simulink model "VehicleDynamicsModel"  (R2018a)
settings: Solver=ode15s  StartTime=0.0  StopTime=12  FixedStep=0.01  RelTol=1e-2  EnableMultiTasking=on
PreLoadFcn:
  | PowerTrain_14DOF_ini
StopFcn:
  | AfterSim
undefined symbols (not defined in the file): AccelCmd2TrqCmd, Chasis, GearRatio, Motor, Motor_J, Motor_RotorDamping, VEH, X, Y, Z
libraries: sm_lib x186, autolibutils x40, nesl_utility x23, vehdynlibtire x4, fuzblock x3, sharedtransform x2, autolibmappedmotorcommon x2, vehdynlibeom x1, vehdynlibsuspension x1, simulink x1, vehdynlibsteering x1
(part 5 of 11)

== system VehicleDynamicsModel/E23/PowerTrain/PowerTrain/MotorRL/Motor/Motor ==
  TrqCmd : Inport
  BattVolt : Inport  Port=2
  MtrSpd : Inport  Port=3
  Bus Creator : BusCreator  Inputs=3
  Bus Selector : BusSelector  OutputSignals=signal1.MechPwr,BattCur,MtrTrq
  Divide : Product  Inputs=**
  Mapped Motor : Subsystem  AncestorBlock=autolibmappedmotor/Mapped Motor  mask(MappedMotor){port_config=Speed, param_by=Tabulated torque-speed envelope, w_t=Motor.Motor_n, T_t=Motor.Motor_Tq, torque_max=123, power_max=50, Tc=Motor.Motor_Tc, param_loss=Tabulated efficiency data, eff=96, w_eff=1000, T_eff=120, Piron=0, Pbase=5, w_eff_bp=Motor.Motor_n_e, T_eff_bp=Motor.Motor_Tq_e, losses_table=[1.49 1.67 2.21 3.10; 0.42 0.69 1.14 2.03; 0.06 0.24 0.78 1.68; 0.42 0.69 1.14 2.03; 1.49 1.67 2.21 3.10], efficiency_table=Motor.Motor_efficiency, J=Motor_J, b=Motor_RotorDamping, omega_o=0, T_t_extended=[0 48.13 49.32 50.18 50.79 51.89 53.34 54.25 55.67 57.12 58.37 60.15 61.25 63.29 65.1 66.47 68.15 70.26 72.09 75.05 77 80.33 82 85.17 88.15 92.06 96.45 99.14 104.15 109.88 114.54 119.13 120.12 120.08 120.05 120 120.16 120.38 120.32 120.12 120.03 120.29 120.06 120.09 120.09 120 120.12 120.08 120.17 120.13 120.02 120.13 120.17 120.08 120.12 120 120.09 120.09 120.06 120.29 120.03 120.12 120.32 120.38 120.16 120 120.05 120.08 120.12 119.13 114.54 109.88 104.15 99.14 96.45 92.06 88.15 85.17 82 80.33 77 75.05 72.09 70.26 68.15 66.47 65.1 63.29 61.25 60.15 58.37 57.12 55.67 54.25 53.34 51.89 50.79 50.18 49.32 48.13 0], w_t_extended=[-1047.1975511966 -1026.14888041755 -1005.30964914873 -984.365698124802 -963.42174710087 -942.373076321818 -921.533845053006 -900.485174273954 -879.645943005142 -858.70199198121 -837.758040957278 -816.918809688466 -795.870138909414 -774.821468130363 -753.877517106431 -733.038285837618 -712.094334813686 -691.150383789755 -670.206432765823 -649.26248174189 -628.318530717959 -607.374579694027 -586.325908914975 -565.486677646163 -544.542726622231 -523.598775598299 -502.550104819247 -481.710873550435 -460.766922526503 -439.718251747451 -418.879020478639 -416.784625376246 -397.935069454707 -376.886398675656 -356.151887161963 -335.103216382911 -314.159265358979 -293.215314335047 -251.327412287183 -230.383461263251 -209.43951023932 -188.495559215388 -167.551608191456 -146.607657167524 -125.663706143592 -104.71975511966 -83.7758040957278 -62.8318530717959 -41.8879020478639 -20.943951023932 0 20.943951023932 41.8879020478639 62.8318530717959 83.7758040957278 104.71975511966 125.663706143592 146.607657167524 167.551608191456 188.495559215388 209.43951023932 230.383461263251 251.327412287183 293.215314335047 314.159265358979 335.103216382911 356.151887161963 376.886398675656 397.935069454707 416.784625376246 418.879020478639 439.718251747451 460.766922526503 481.710873550435 502.550104819247 523.598775598299 544.542726622231 565.486677646163 586.325908914975 607.374579694027 628.318530717959 649.26248174189 670.206432765823 691.150383789755 712.094334813686 733.038285837618 753.877517106431 774.821468130363 795.870138909414 816.918809688466 837.758040957278 858.70199198121 879.645943005142 900.485174273954 921.533845053006 942.373076321818 963.42174710087 984.365698124802 1005.30964914873 1026.14888041755 1047.1975511966], KLossIron=0, KLossCopper=0.34687, x_w_eff_vec=[-1047.1975511966 -1026.25360017267 -1005.30964914873 -984.365698124802 -963.42174710087 -942.477796076938 -921.533845053006 -900.589894029074 -879.645943005142 -858.70199198121 -837.758040957278 -816.814089933346 -795.870138909414 -774.926187885482 -753.98223686155 -733.038285837618 -712.094334813686 -691.150383789755 -670.206432765823 -649.262481741891 -628.318530717959 -607.374579694027 -586.430628670095 -565.486677646163 -544.542726622231 -523.598775598299 -502.654824574367 -481.710873550435 -460.766922526503 -439.822971502571 -418.879020478639 -397.935069454707 -376.991118430775 -356.047167406843 -335.103216382911 -314.159265358979 -293.215314335047 -272.271363311115 -251.327412287183 -230.383461263251 -209.43951023932 -188.495559215388 -167.551608191456 -146.607657167524 -125.663706143592 -104.71975511966 -83.7758040957278 -62.8318530717959 -41.8879020478639 -20.943951023932 0 20.943951023932 41.8879020478639 62.8318530717959 83.7758040957278 104.71975511966 125.663706143592 146.607657167524 167.551608191456 188.495559215388 209.43951023932 230.383461263251 251.327412287183 272.271363311115 293.215314335047 314.159265358979 335.103216382911 356.047167406843 376.991118430775 397.935069454707 418.879020478639 439.822971502571 460.766922526503 481.710873550435 502.654824574367 523.598775598299 544.542726622231 565.486677646163 586.430628670095 607.374579694027 628.318530717959 649.262481741891 670.206432765823 691.150383789755 712.094334813686 733.038285837618 753.98223686155 774.926187885482 795.870138909414 816.814089933346 837.758040957278 858.70199198121 879.645943005142 900.589894029074 921.533845053006 942.477796076938 963.42174710087 984.365698124802 1005.30964914873 1026.25360017267 1047.1975511966], x_T_eff_vec=[-120 -115 -110 -105 -100 -95 -90 -85 -80 -75 -70 -65 -60 -55 -50 -45 -40 -35 -30 -25 -20 -15 -10 -5 0 5 10 15 20 25 30 35 40 45 50 55 60 65 70 75 80 85 90 95 100 105 110 115 120], x_losses_mat=[125538042.437448 120307290.669221 115076538.900994 109845787.132767 104615035.36454 99384283.5963131 94153531.8280861 88922780.0598591 83692028.2916321 78461276.5234051 73230524.7551781 67999772.9869511 62769021.2187241 8077.86936584377 6537.62250747031 5294.23011144442 3494.44036585647 3669.22354297158 2256.0204479155 2432.01617081177 2071.37977159766 1610.62908921637 1294.28910822051 2661.42967385561 0 1764.52787376627 1151.91730631626 1460.84058391925 1884.95559215388 2225.29479629277 2104.86707790516 3335.32420056116 3225.36845768552 4759.51287018854 5811.94640914111 7084.29143384498 62769.0212187241 67999.7729869511 73230.5247551781 78461.2765234051 83692.0282916321 88922.7800598591 94153.5318280861 99384.2835963131 104615.03536454 109845.787132767 115076.538900994 120307.290669221 125538.042437448;123027281.588699 117901144.855837 112775008.122974 107648871.390112 102522734.657249 97396597.9243868 92270461.1915244 87144324.4586619 82018187.7257994 76892050.992937 71765914.2600745 66639777.5272121 61513640.7943496 7478.98291858562 6148.32783978025 4960.79398090109 3813.40135583285 3038.69016103186 2786.66462860407 2322.22052383673 1712.27577926967 1559.72463462365 1426.00158566133 1227.18057517549 0 990.334724166622 1252.02939221065 1416.22996823828 1580.4305442659 2129.47622035828 2555.37146442994 2801.67232847138 3489.26224058706 4479.59696475368 5490.45676092376 6603.9419171111 61513.6407943496 66639.777527212 71765.9142600745 76892.050992937 82018.1877257994 87144.3244586619 92270.4611915244 97396.5979243868 102522.734657249 107648.871390112 112775.008122974 117901.144855837 123027.281588699;120516520.73995 115494999.042452 110473477.344954 105451955.647456 100430433.949959 95408912.2524606 90387390.5549626 85365868.8574647 80344347.1599668 75322825.4624689 70301303.7649709 65279782.067473 60258260.3699751 55236738.6724772 6085.95527511565 4419.61047732237 3213.51680505427 2811.82720442249 2586.95316881922 1949.95406084884 1819.86261459858 1582.94613263751 1255.2235214343 1073.63166413942 0 884.672491250885 1115.89371055509 1432.56625003695 1668.8140175869 1809.55736846772 2382.5838684825 2603.75199129522 2975.71656148025 4026.26514484068 5428.67210540316 55236.7386724772 60258.2603699751 65279.782067473 70301.3037649709 75322.8254624689 80344.3471599668 85365.8688574647 90387.3905549627 95408.9122524606 100430.433949959 105451.955647456 110473.477344954 115494.999042452 120516.52073995;118005759.891201 113088853.229068 108171946.566934 103255039.904801 98338133.2426677 93421226.5805343 88504319.9184009 83587413.2562675 78670506.5941342 73753599.9320008 68836693.2698674 63919786.607734 59002879.9456006 6555.08099423915 5226.72052101664 4009.3848227875 2647.3869362588 2673.06202508028 2394.40304949276 2110.88192594624 1596.26869966184 1424.73982623326 1266.56534521701 958.492286704556 0 802.258043971713 1122.17689586227 1299.36272152474 1476.5485471872 1944.12225379649 2214.8228207808 2480.6015592745 2480.6015592745 3676.60588249613 4724.95535099905 5847.13224686132 59002.8799456006 63919.786607734 68836.6932698674 73753.5999320008 78670.5065941342 83587.4132562676 88504.3199184009 93421.2265805343 98338.1332426677 103255.039904801 108171.946566934 113088.853229068 118005.759891201;115494999.042452 110682707.415683 105870415.788915 101058124.162146 96245832.5353769 91433540.9086081 86621249.2818392 81808957.6550704 76996666.0283015 72184374.4015327 67372082.7747638 62559791.147995 6494.25560337182 6018.70378756779 4590.23504916625 3616.74577866145 2723.1621117198 2694.66773757155 2276.04490415416 1840.76813897098 1517.36326943611 1308.02625424273 1178.59675010095 1036.00029913034 0 852.62824618427 1050.12970433995 1199.46007514058 1406.59575076727 1710.07360110404 2109.8936261509 2495.26232499125 2543.43341234629 3338.25635370451 4190.88459988878 5404.79600123588 5838.33578743127 62559.791147995 67372.0827747638 72184.3744015327 76996.6660283015 81808.9576550704 86621.2492818392 91433.5409086081 96245.8325353769 ...(+77378 chars)], aMode=1}
      mask prompts: port_config "autoblks_shared:autoblkpbgenericelectricmachine:blkPrm_port_config"; param_by "autoblks_shared:autoblkpbgenericelectricmachine:blkPrm_param_by"; w_t "autoblks_shared:autoblkpbgenericelectricmachine:blkPrm_w_t"; T_t "autoblks_shared:autoblkpbgenericelectricmachine:blkPrm_T_t"; torque_max "autoblks_shared:autoblkpbgenericelectricmachine:blkPrm_torque_max"; power_max "autoblks_shared:autoblkpbgenericelectricmachine:blkPrm_power_max"; Tc "autoblks_shared:autoblkpbgenericelectricmachine:blkPrm_Tc"; param_loss "autoblks_shared:autoblkpbgenericelectricmachine:blkPrm_param_loss"; eff "autoblks_shared:autoblkpbgenericelectricmachine:blkPrm_eff"; w_eff "autoblks_shared:autoblkpbgenericelectricmachine:blkPrm_w_eff"; T_eff "autoblks_shared:autoblkpbgenericelectricmachine:blkPrm_T_eff"; Piron "autoblks_shared:autoblkpbgenericelectricmachine:blkPrm_Piron"; Pbase "autoblks_shared:autoblkpbgenericelectricmachine:blkPrm_Pbase"; w_eff_bp "autoblks_shared:autoblkpbgenericelectricmachine:blkPrm_w_eff_bp"; T_eff_bp "autoblks_shared:autoblkpbgenericelectricmachine:blkPrm_T_eff_bp"; losses_table "autoblks_shared:autoblkpbgenericelectricmachine:blkPrm_losses_table"; efficiency_table "autoblks_shared:autoblkpbgenericelectricmachine:blkPrm_efficiency_table"; J "autoblks_shared:autoblkpbgenericelectricmachine:blkPrm_J"; b "autoblks_shared:autoblkpbgenericelectricmachine:blkPrm_b"; omega_o "autoblks_shared:autoblkpbgenericelectricmachine:blkPrm_omega_o"; T_t_extended "autoblks_shared:autoblkpbgenericelectricmachine:blkPrm_T_t_extended"; w_t_extended "autoblks_shared:autoblkpbgenericelectricmachine:blkPrm_w_t_extended"; KLossIron "autoblks_shared:autoblkpbgenericelectricmachine:blkPrm_KLossIron"; KLossCopper "autoblks_shared:autoblkpbgenericelectricmachine:blkPrm_KLossCopper"; x_w_eff_vec "autoblks_shared:autoblkpbgenericelectricmachine:blkPrm_x_w_eff_vec"; x_T_eff_vec "autoblks_shared:autoblkpbgenericelectricmachine:blkPrm_x_T_eff_vec"; x_losses_mat "autoblks_shared:autoblkpbgenericelectricmachine:blkPrm_x_losses_mat"
      mask help: autoblks_shared:autoblkpbgenericelectricmachine:blkDesc
      mask init:
      | autosharedicon('pbgenericelectricmachine',gcb,'Initialization');
      mask Help: eval('autosharedhelp(''pbgenericelectricmachine'')');
      mask TypeOptions port_config: autoblks_shared:autoblkpbgenericelectricmachine:blkCmb_port_configTorque | autoblks_shared:autoblkpbgenericelectricmachine:blkCmb_port_configSpeed
      mask Callback port_config: autosharedicon('pbgenericelectricmachine', gcb, 'PortConfig');
      mask TypeOptions param_by: autoblks_shared:autoblkpbgenericelectricmachine:blkCmb_param_byTabulatedtorquespeedenvelope | autoblks_shared:autoblkpbgenericelectricmachine:blkCmb_param_byMaximumtorqueandpower
      mask Callback param_by: autosharedicon('pbgenericelectricmachine', gcb, 'ElectricalTorque');
      mask TypeOptions param_loss: autoblks_shared:autoblkpbgenericelectricmachine:blkCmb_param_lossSingleefficiencymeasurement | autoblks_shared:autoblkpbgenericelectricmachine:blkCmb_param_lossTabulatedlossdata | autoblks_shared:autoblkpbgenericelectricmachine:blkCmb_param_lossTabulatedefficiencydata
      mask Callback param_loss: autosharedicon('pbgenericelectricmachine', gcb, 'ElectricalLoss');
      mask DialogControl BlockOptions Prompt: autoblks_shared:autoblkpbgenericelectricmachine:blkDlg_BlockOptions
      mask DialogControl port_config Prompt: Port configuration:
      mask DialogControl ParameterGroupVar Prompt: autoblks_shared:autoblkpbgenericelectricmachine:blkDlg_ParameterGroupVar
      mask DialogControl ElectricalTorque Prompt: autoblks_shared:autoblkpbgenericelectricmachine:blkDlg_ElectricalTorque
      mask DialogControl param_by Prompt: Parameterized by:
      mask DialogControl w_t Prompt: Vector of rotational speeds, w_t [rad/s]:
      mask DialogControl T_t Prompt: Vector of maximum torque values, T_t, [Nm]:
      mask DialogControl torque_max Prompt: Maximum torque, torque_max [Nm]:
      mask DialogControl power_max Prompt: Maximum power, power_max [W]:
      mask DialogControl Tc Prompt: Torque control time constant, Tc, [s]:
      mask DialogControl ElectricalLosses Prompt: autoblks_shared:autoblkpbgenericelectricmachine:blkDlg_ElectricalLosses
      mask DialogControl param_loss Prompt: Parameterize losses by:
      mask DialogControl eff Prompt: Motor and drive overall efficiency, eff [%]:
      mask DialogControl w_eff Prompt: Speed at which efficiency is measured, w_eff, [rad/s]:
      mask DialogControl T_eff Prompt: Torque at which efficiency is measured, T_eff, [Nm]:
      mask DialogControl Piron Prompt: Iron losses, Piron [W]:
      mask DialogControl Pbase Prompt: Fixed losses independent of torque and speed, Pbase [W]:
      mask DialogControl w_eff_bp Prompt: Vector of speeds (w) for tabulated losses, w_eff_bp [rad/s]:
      mask DialogControl T_eff_bp Prompt: Vector of torques (T) for tabulated losses, T_eff_bp [Nm]:
      mask DialogControl losses_table Prompt: Corresponding losses, losses_table [W]:
      mask DialogControl efficiency_table Prompt: Corresponding efficiency, efficiency_table [%]:
      mask DialogControl Mechanical Prompt: autoblks_shared:autoblkpbgenericelectricmachine:blkDlg_Mechanical
      mask DialogControl J Prompt: Rotor inertia, J [kg*m^2]:
      mask DialogControl b Prompt: Rotor damping, b [N*m*s/rad]:
      mask DialogControl omega_o Prompt: Initial rotor speed, omega_o [rad/s]:
      mask DialogControl T_t_extended Prompt: Tabulated Torque Extended:
      mask DialogControl w_t_extended Prompt: Tabulated Speed  Extended:
      mask DialogControl KLossIron Prompt: Single Efficiency Iron Loss:
      mask DialogControl KLossCopper Prompt: Single Efficiency Copper Loss:
      mask DialogControl x_w_eff_vec Prompt: Tabulated Speed Power Loss:
      mask DialogControl x_T_eff_vec Prompt: Tabulated Torque Power Loss:
      mask DialogControl x_losses_mat Prompt: Tabulated Speed Power Loss:
      mask Display:
      | IconInfo = autosharedicon('pbgenericelectricmachine', gcb, 'DrawCommands');
      | 
      | image(IconInfo.image, IconInfo.position);
      | 
      | for i = 1:numel(IconInfo.lconn)
      |     port_label('lconn', i, IconInfo.lconn{i})
      | end
      | 
      | for j = 1:numel(IconInfo.rconn)
      |     port_label('rconn', j, IconInfo.rconn{j})
      | end
      | 
      | for k = 1:numel(IconInfo.input)
      |     port_label('input', k, IconInfo.input{k})
      | end
      | 
      | for m = 1:numel(IconInfo.output)
      |     port_label('output', m, IconInfo.output{m})
      | end
  MechPwr : Outport
  BattCurr : Outport  Port=2
  MtrTrq : Outport  Port=3
  P_in : Outport  Port=4
  wires:
  TrqCmd/1 -> Mapped Motor/3(TrqCmd)
  Bus Selector/3 -> MtrTrq/1  "<MtrTrq>"
  Bus Selector/2 -> BattCurr/1, Divide/2  "<BattCur>"
  Mapped Motor/3(MtrTrq) -> Bus Creator/3  "MtrTrq"
  Mapped Motor/1(Info) -> Bus Creator/1
  BattVolt/1 -> Mapped Motor/1(BattVolt), Divide/1
  Mapped Motor/2(BattCurr) -> Bus Creator/2  "BattCur"
  Bus Creator/1 -> Bus Selector/1
  Bus Selector/1 -> MechPwr/1  "<MechPwr>"
  Divide/1 -> P_in/1
  MtrSpd/1 -> Mapped Motor/2(MtrSpd)
